simulink model "Observador_Estados"  (R2016a)
settings: Solver=VariableStepAuto  StartTime=0.0  StopTime=10.0  RelTol=1e-3
values from neighbouring files (symbols this model uses):
  ki = kt(:,3:3)    [ejemplodiscretro.m]
  kp = kt(:,1:2)    [ejemplodiscretro.m]
undefined symbols (not defined in the file or in its folder): A, B, C, h
settings Model: Creator=Daniel  LastModifiedBy=Daniel

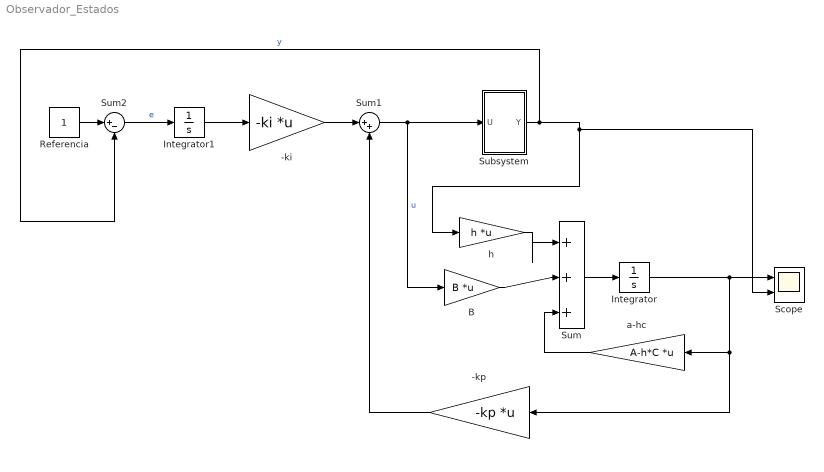
== system Observador_Estados ==
  -ki : Gain  Gain=-ki  Multiplication=Matrix(K*u) (u vector)
  -kp : Gain  Gain=-kp  Multiplication=Matrix(K*u) (u vector)
  B : Gain  Gain=B  Multiplication=Matrix(K*u) (u vector)
  Integrator : Integrator
  Integrator1 : Integrator
  Referencia : Constant
  Scope : Scope  NumInputPorts=2
  Subsystem : Subsystem
  Sum : Sum  Inputs=|+++
  Sum1 : Sum  Inputs=|++
  Sum2 : Sum  Inputs=|+-
  a-hc : Gain  Gain=A-h*C  Multiplication=Matrix(K*u) (u vector)
  h : Gain  Gain=h  Multiplication=Matrix(K*u) (u vector)
  wires:
  Sum/1 -> Integrator/1
  a-hc/1 -> Sum/3
  B/1 -> Sum/2
  h/1 -> Sum/1
  Subsystem/1(Y) -> Scope/2, h/1, Sum2/2  "y"
  Sum1/1 -> Subsystem/1(U), B/1  "u"
  Integrator1/1 -> -ki/1
  Sum2/1 -> Integrator1/1  "e"
  Referencia/1 -> Sum2/1
  -ki/1 -> Sum1/1
  Integrator/1 -> Scope/1, -kp/1, a-hc/1
  -kp/1 -> Sum1/2

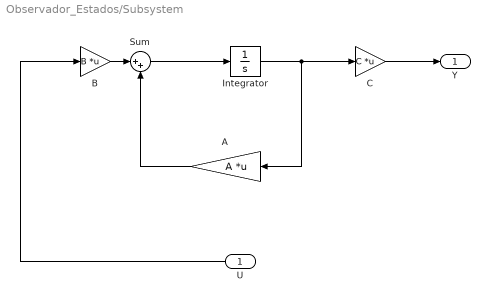
== system Observador_Estados/Subsystem ==
  U : Inport
  A : Gain  Gain=A  Multiplication=Matrix(K*u) (u vector)
  B : Gain  Gain=B  Multiplication=Matrix(K*u) (u vector)
  C : Gain  Gain=C  Multiplication=Matrix(K*u) (u vector)
  Integrator : Integrator
  Sum : Sum  Inputs=|++
  Y : Outport
  wires:
  Sum/1 -> Integrator/1
  A/1 -> Sum/2
  U/1 -> B/1
  B/1 -> Sum/1
  C/1 -> Y/1
  Integrator/1 -> A/1, C/1
